simulink model "geometria_schemat"  (R2022b)
settings: Solver=VariableStepAuto  StartTime=0.0  StopTime=10.0  RelTol=1e-3
undefined symbols (not defined in the file): delta, delta_dyn, delta_h, Q, V
settings Model: Creator=julia  LastModifiedBy=lukas

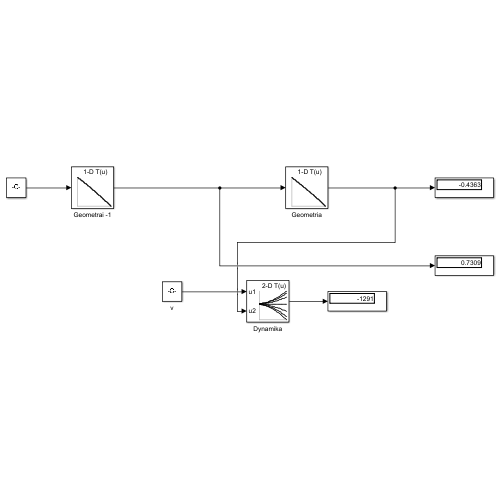
[thumbnail: Simulink's stored preview of the top-level diagram]
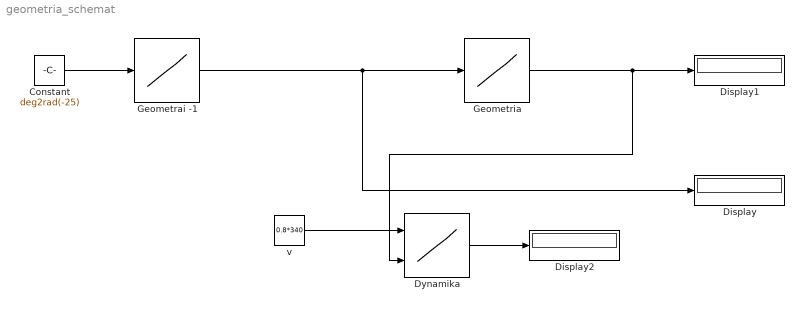
== system geometria_schemat ==
  Constant : Constant  Value=deg2rad(-25)
  Display : Display
  Display1 : Display
  Display2 : Display
  Dynamika : Lookup_n-D  BreakpointsForDimension1=V  BreakpointsForDimension2=delta_dyn  Table=Q  InternalRulePriority=Speed  RndMeth=Simplest
      settings: InputPortMap=u0,u1
  Geometrai -1 : Lookup_n-D  NumberOfTableDimensions=1  BreakpointsForDimension1=delta  Table=delta_h  InternalRulePriority=Speed  RndMeth=Simplest
  Geometria : Lookup_n-D  NumberOfTableDimensions=1  BreakpointsForDimension1=flip(delta_h)  Table=flip(delta)  InternalRulePriority=Speed  RndMeth=Simplest
  v : Constant  Value=0.8*340
  wires:
  Geometrai -1/1 -> Display/1, Geometria/1
  Geometria/1 -> Dynamika/2, Display1/1
  Constant/1 -> Geometrai -1/1
  Dynamika/1 -> Display2/1
  v/1 -> Dynamika/1
